simulink model "MPC_MMC_qudratic_paper_v1v7"  (R2019b)
settings: Solver=ode3  StartTime=0.0  StopTime=3  FixedStep=0.000080  RelTol=1e-3  EnableMultiTasking=on
settings Model: Creator=cary  LastModifiedBy=adshetgaonkar
settings DataIOCC: LimitDataPoints=on  SaveFormat=Array  SignalLoggingSaveFormat=ModelDataLogs  ReturnWorkspaceOutputs=off
settings OptimizationCC: ExpressionDepthLimit=2147483647  LifeSpan=1  EfficientTunableParamExpr=on
settings DebuggingCC: UnderspecifiedInitializationDetection=Classic  MergeDetectMultiDrivingBlocksExec=none  SolverPrmCheckMsg=warning  FcnCallInpInsideContextMsg=warning  StateNameClashWarn=warning  SFUnexpectedBacktrackingDiag=warning  SFNoUnconditionalDefaultTransitionDiag=warning  SFExecutionAtInitializationDiag=none  ArithmeticOperatorsInVariantConditions=warning
settings HardwareCC: ProdBitPerPointer=32  ProdBitPerSizeT=32  ProdBitPerPtrDiffT=32  ProdLargestAtomicFloat=None  ProdIntDivRoundTo=Undefined  ProdEndianess=Unspecified  ProdWordSize=32  ProdHWDeviceType=32-bit Generic
settings ModelReferenceCC: PropagateSignalLabelsOutOfModel=off
settings SFSimCC: SimUseLocalCustomCode=off  MATLABDynamicMemAlloc=off  CustomCodeUndefinedFunction=UseInterfaceOnly
settings RTWCC: SystemTargetFile=ert.tlc  TemplateMakefile=ert_default_tmf  RTWUseLocalCustomCode=off
settings CodeAppCC: IgnoreCustomStorageClasses=off  CustomSymbolStrType=$N$R$M  StateflowObjectComments=on  InternalIdentifier=Classic
settings ERTTargetCC: MultiwordLength=2048  GenerateSampleERTMain=on  IncludeMdlTerminateFcn=off  SupportComplex=off  SupportContinuousTime=on  ERTCustomFileTemplate=example_file_process.tlc  ConvertIfToSwitch=off  SuppressUnreachableDefaultCases=off
settings ConfigComp: CovMetricSettings=dw  CovHtmlReporting=on  CovSaveCumulativeToWorkspaceVar=on  CovSaveSingleToWorkspaceVar=on  CovExternalEMLEnable=off

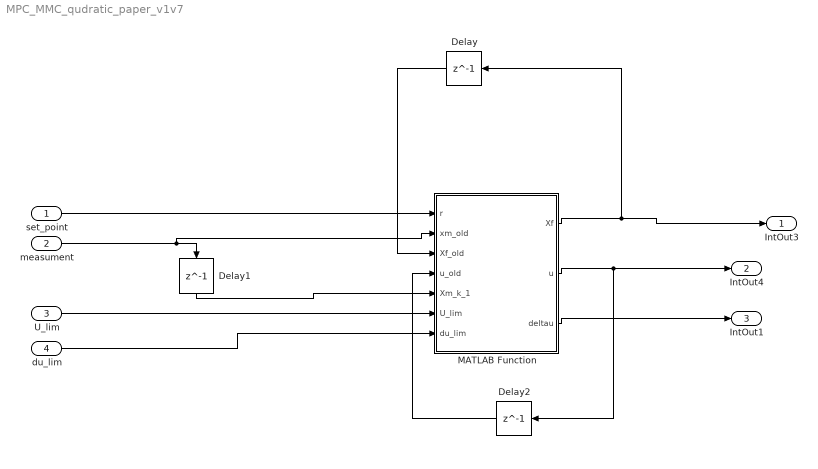
== system MPC_MMC_qudratic_paper_v1v7 ==
  set_point : Inport  PortDimensions=5
  measument : Inport  Port=2  PortDimensions=5
  U_lim : Inport  Port=3  PortDimensions=5
  du_lim : Inport  Port=4  PortDimensions=5
  Delay : Delay  DelayLength=1
  Delay1 : Delay  DelayLength=1
  Delay2 : Delay  DelayLength=1
  MATLAB Function : MATLAB Function  TreatAsAtomicUnit=on
  IntOut3 : Outport  SignalName=Xf
  IntOut4 : Outport  Port=2  SignalName=u
  IntOut1 : Outport  Port=3  SignalName=delta_u
  wires:
  set_point/1 -> MATLAB Function/1(r)
  MATLAB Function/1(Xf) -> Delay/1, IntOut3/1
  measument/1 -> MATLAB Function/2(xm_old), Delay1/1
  MATLAB Function/3(deltau) -> IntOut1/1
  Delay1/1 -> MATLAB Function/5(Xm_k_1)
  Delay/1 -> MATLAB Function/3(Xf_old)
  Delay2/1 -> MATLAB Function/4(u_old)
  MATLAB Function/2(u) -> Delay2/1, IntOut4/1
  U_lim/1 -> MATLAB Function/6(U_lim)
  du_lim/1 -> MATLAB Function/7(du_lim)

== matlab function MPC_MMC_qudratic_paper_v1v7/MATLAB Function ==
  data: r input; Xf output; xm_old input; u output; Xf_old input; u_old input; Xm_k_1 input; deltau output; U_lim input; du_lim input
function [Xf,u,deltau] = fcn(r,xm_old,Xf_old,u_old,Xm_k_1,U_lim,du_lim)
D = []; 
D= coder.load('initial_qudratic_papervx.mat'); 
gamma=[(U_lim - u_old);(U_lim + u_old); du_lim; du_lim];
eta = QPhild(D.Omega,D.Psi*(D.Xf+Xf_old),D.M,gamma);
%eta= -(D.Omega\D.Psi)*(D.Xf+Xf_old);
deltau= D.Lzerot*eta;
u=D.up+u_old+deltau;
y = xm_old;
xm = xm_old;
y_delta_k=y-Xm_k_1;
Xf=[y_delta_k;y-r];
end
